simulink model "KD_cl_harness_cl_ouports_added"  (R2015b)
settings: Solver=ode45  StartTime=0  StopTime=inf  FixedStep=0.01  MaxStep=0.005  RelTol=1e-5  AbsTol=1e-5
undefined symbols (not defined in the file or in its folder): A2, bin_vec, c_0, c_1000, c_1000inv, c_100inv, c_1d2p4, c_1p7, c_4400inv, c_5500inv, c_80, c_compmap, c_ctok, c_fflow_max, c_fflow_min, c_filt, c_flowdiv, c_flowmin, c_flowmult, c_inf, c_km1d2k, c_n1, c_p00001, c_p01, c_p1e9, c_p4d1p4, c_pincomp, c_rair, c_roacorr, c_rpmtoradpers, c_svrthrottle1, c_svrthrottle2, c_svrthrottlearg, c_svrthrottlebeta, c_vnliftmax, c_vnliftmin, cl_offset, clff, Coefs, const, const_exhat, const_vec, Dual_array, dual_zero, egr_ecu_ff, expcon, f_mat, gs_jul, HQP_eps, HQP_INF, HQP_saturation, IV, L2, length_L, maxL, mHQP_saturation, minL, Newton, nRed, num_constraints ... (+22)
libraries: simulink x33
(part 3 of 6)

== system KD_cl_harness_cl_ouports_added/ctrl_rb_explicit_20140220_v6_simp/egr_est ==
  maf : Inport
  wcyl : Inport  Port=2
  ene : Inport  Port=3
  valve : Inport  Port=4
  Gain7 : Gain  Gain=100
      settings: AttributesFormatString=%<Gain>
  Product3 : Product  Inputs=**/  RndMeth=Zero
  Product4 : Product  Inputs=*/  RndMeth=Zero
  Saturation1 : Saturate  UpperLimit=c_inf  LowerLimit=c_0
      settings: AttributesFormatString=%<LowerLimit>\n%<UpperLimit>
  Saturation3 : Saturate  UpperLimit=c_inf  LowerLimit=c_p00001
      settings: AttributesFormatString=%<LowerLimit>\n%<UpperLimit>
  Sum11 : Sum  Inputs=+-|
  custom_filter : Subsystem  Tag=FilterWizardSubSystem
      settings: ErrorFcn=dspFilterRealizedInBasicElemsAlgLoopErrFcnCallback
  interp : Subsystem  Tag=FilterWizardSubSystem
      settings: ErrorFcn=dspFilterRealizedInBasicElemsAlgLoopErrFcnCallback
  mintos : Constant  Value=60  OutDataTypeStr=single
      settings: AttributesFormatString=%<Value>
  egrr : Outport
  wegr : Outport  Port=2
  wcylgps : Outport  Port=3
  sat_out-17 : Outport  Port=4
  sat_out-18 : Outport  Port=5
  sat_out-25 : Outport  Port=6
  sat_out-26 : Outport  Port=7
  wires:
  [MAF] -> Sum11/2
  Product3/1 -> interp/3(Wcyl)
  mintos/1 -> Product3/3
  Sum11/1 -> Saturation1/1, sat_out-17/1
  Product4/1 -> Gain7/1
  Gain7/1 -> egrr/1
  maf/1 -> [MAF]
  wcyl/1 -> Product3/1
  ene/1 -> Product3/2
  Saturation1/1 -> custom_filter/1(Input)
  Saturation3/1 -> Product4/2
  interp/1(Wcylhat) -> wcylgps/1, Sum11/1, [wcyl]
  [MAF] -> interp/2(MAF)
  valve/1 -> interp/1(valve)
  custom_filter/1(Output) -> Product4/1, wegr/1
  [wcyl] -> Saturation3/1, sat_out-18/1
  custom_filter/2(sat_out-25) -> sat_out-25/1
  custom_filter/3(sat_out-26) -> sat_out-26/1

== system KD_cl_harness_cl_ouports_added/ctrl_rb_explicit_20140220_v6_simp/gain_schechule ==
  ene : Inport
  qv : Inport  Port=2
  maprefadd1 : Lookup2D  RowIndex=gs_jul.rowsene  ColumnIndex=gs_jul.colsqv  Table=gs_jul.vegr  LookUpMeth=Interpolation-Use End Values
      settings: AttributesFormatString=%<LookUpMeth>\n%<RowIndex>\n%<ColumnIndex>\n%<Table>
  maprefadd2 : Lookup2D  RowIndex=gs_jul.rowsene  ColumnIndex=gs_jul.colsqv  Table=gs_jul.vgt  LookUpMeth=Interpolation-Use End Values
      settings: AttributesFormatString=%<LookUpMeth>\n%<RowIndex>\n%<ColumnIndex>\n%<Table>
  zero1 : Constant  Value=0  OutDataTypeStr=single  SampleTime=sample_time
      settings: AttributesFormatString=%<Value>\n%<SampleTime>
  zero15 : Constant  Value=0  OutDataTypeStr=single  SampleTime=sample_time
      settings: AttributesFormatString=%<Value>\n%<SampleTime>
  gs1 : Outport
  gs2 : Outport  Port=2
  gs3 : Outport  Port=3
  gs4 : Outport  Port=4
  wires:
  qv/1 -> [w_f]
  ene/1 -> [engine_speed_rpm]
  zero1/1 -> gs4/1
  zero15/1 -> gs3/1
  maprefadd1/1 -> gs2/1
  maprefadd2/1 -> gs1/1
  [engine_speed_rpm] -> maprefadd1/1
  [w_f] -> maprefadd1/2
  [engine_speed_rpm] -> maprefadd2/1
  [w_f] -> maprefadd2/2

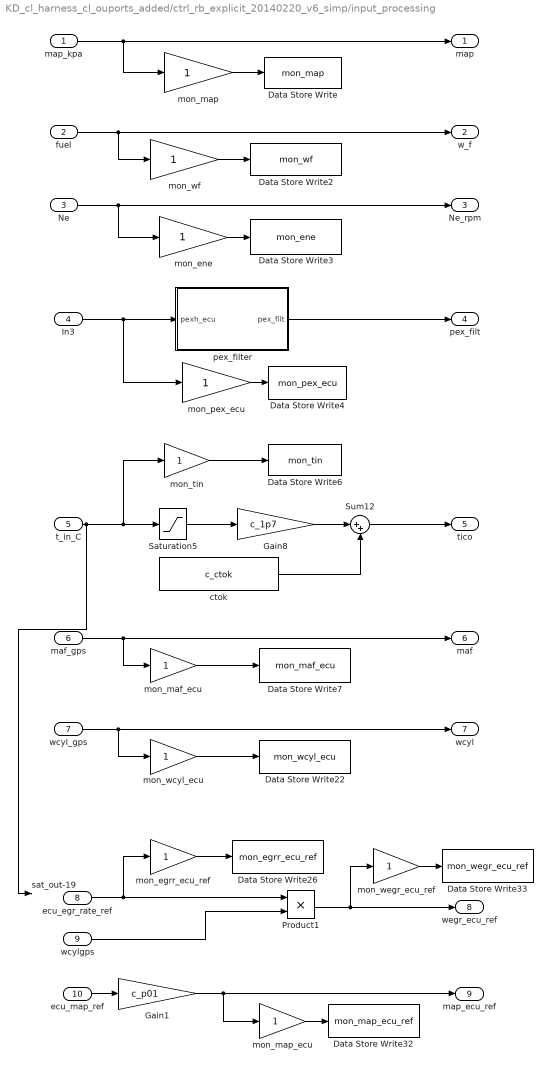
== system KD_cl_harness_cl_ouports_added/ctrl_rb_explicit_20140220_v6_simp/input_processing ==
  map_kpa : Inport
  fuel : Inport  Port=2
  Ne : Inport  Port=3
  In3 : Inport  Port=4
  t_in_C : Inport  Port=5
  maf_gps : Inport  Port=6
  wcyl_gps : Inport  Port=7
  ecu_egr_rate_ref : Inport  Port=8
  wcylgps : Inport  Port=9
  ecu_map_ref : Inport  Port=10
  Data Store Write : DataStoreWrite  DataStoreName=mon_map
  Data Store Write2 : DataStoreWrite  DataStoreName=mon_wf
  Data Store Write22 : DataStoreWrite  DataStoreName=mon_wcyl_ecu
  Data Store Write26 : DataStoreWrite  DataStoreName=mon_egrr_ecu_ref
  Data Store Write3 : DataStoreWrite  DataStoreName=mon_ene
  Data Store Write32 : DataStoreWrite  DataStoreName=mon_map_ecu_ref
  Data Store Write33 : DataStoreWrite  DataStoreName=mon_wegr_ecu_ref
  Data Store Write4 : DataStoreWrite  DataStoreName=mon_pex_ecu
  Data Store Write6 : DataStoreWrite  DataStoreName=mon_tin
  Data Store Write7 : DataStoreWrite  DataStoreName=mon_maf_ecu
  Gain1 : Gain  Gain=c_p01
      settings: AttributesFormatString=%<Gain>
  Gain8 : Gain  Gain=c_1p7
      settings: AttributesFormatString=%<Gain>
  Product1 : Product  RndMeth=Zero
  Saturation5 : Saturate  UpperLimit=c_inf  LowerLimit=c_0
      settings: AttributesFormatString=%<LowerLimit>\n%<UpperLimit>
  Sum12 : Sum  Inputs=|++
  ctok : Constant  Value=c_ctok  OutDataTypeStr=single  SampleTime=sample_time
      settings: AttributesFormatString=%<Value>\n%<SampleTime>
  mon_egrr_ecu_ref : Gain
  mon_ene : Gain
  mon_maf_ecu : Gain
  mon_map : Gain
  mon_map_ecu : Gain
  mon_pex_ecu : Gain
  mon_tin : Gain
  mon_wcyl_ecu : Gain
  mon_wegr_ecu_ref : Gain
  mon_wf : Gain
  pex_filter : Subsystem  SystemSampleTime=.016
  map : Outport
  w_f : Outport  Port=2
  Ne_rpm : Outport  Port=3
  pex_filt : Outport  Port=4
  tico : Outport  Port=5
  maf : Outport  Port=6
  wcyl : Outport  Port=7
  wegr_ecu_ref : Outport  Port=8
  map_ecu_ref : Outport  Port=9
  sat_out-19 : Outport  Port=10
  wires:
  Gain1/1 -> mon_map_ecu/1, map_ecu_ref/1
  Product1/1 -> mon_wegr_ecu_ref/1, wegr_ecu_ref/1
  mon_wegr_ecu_ref/1 -> Data Store Write33/1
  mon_map_ecu/1 -> Data Store Write32/1
  ecu_egr_rate_ref/1 -> Product1/1, mon_egrr_ecu_ref/1
  mon_egrr_ecu_ref/1 -> Data Store Write26/1
  In3/1 -> mon_pex_ecu/1, pex_filter/1(pexh_ecu)
  t_in_C/1 -> Saturation5/1, mon_tin/1, sat_out-19/1
  ctok/1 -> Sum12/2
  Gain8/1 -> Sum12/1
  Saturation5/1 -> Gain8/1
  mon_wf/1 -> Data Store Write2/1
  mon_ene/1 -> Data Store Write3/1
  mon_pex_ecu/1 -> Data Store Write4/1
  mon_tin/1 -> Data Store Write6/1
  mon_maf_ecu/1 -> Data Store Write7/1
  mon_wcyl_ecu/1 -> Data Store Write22/1
  fuel/1 -> w_f/1, mon_wf/1
  Ne/1 -> mon_ene/1, Ne_rpm/1
  maf_gps/1 -> mon_maf_ecu/1, maf/1
  wcyl_gps/1 -> wcyl/1, mon_wcyl_ecu/1
  pex_filter/1(pex_filt) -> pex_filt/1
  Sum12/1 -> tico/1
  wcylgps/1 -> Product1/2
  ecu_map_ref/1 -> Gain1/1
  map_kpa/1 -> mon_map/1, map/1
  mon_map/1 -> Data Store Write/1

== system KD_cl_harness_cl_ouports_added/ctrl_rb_explicit_20140220_v6_simp/invert_flow ==
  valve_flow_command : Inport
  ne_rpm : Inport  Port=2
  qv_mm3st : Inport  Port=3
  Saturation1 : Saturate  UpperLimit=150  LowerLimit=c_0
      settings: AttributesFormatString=%<LowerLimit>\n%<UpperLimit>
  d3inv : Lookup_n-D  NumberOfTableDimensions=3  BreakpointsForDimension1=valveinv.wegr_row  BreakpointsForDimension2=valveinv.ene_column  BreakpointsForDimension3=valveinv.fuel_z  Table=valveinv.valve  ExtrapMethod=Clip  UseLastTableValue=on  InputSameDT=on
      settings: AttributesFormatString=%<BreakpointsForDimension1>\n%<BreakpointsForDimension2>\n%<BreakpointsForDimension3>\n%<Table>\n%<UseLastTableValue>\n%<InterpMethod>
  togps : Gain  Gain=c_1000
      settings: AttributesFormatString=%<Gain>
  uvalve : Outport
  sat_out-20 : Outport  Port=2
  wires:
  Saturation1/1 -> uvalve/1
  d3inv/1 -> Saturation1/1, sat_out-20/1
  togps/1 -> d3inv/1
  qv_mm3st/1 -> d3inv/3
  ne_rpm/1 -> d3inv/2
  valve_flow_command/1 -> togps/1

== system KD_cl_harness_cl_ouports_added/ctrl_rb_explicit_20140220_v6_simp/ntremap ==
  u_EGR_throttle : Inport
  omega_engine_rpm : Inport  Port=2
  T_out_IC : Inport  Port=3
  maf : Inport  Port=4
  Data Store Read18 : DataStoreRead  DataStoreName=man_ntcons
  Divide6 : Product  Inputs=*/
  Saturation1 : Saturate  UpperLimit=50  LowerLimit=8
      settings: AttributesFormatString=%<LowerLimit>\n%<UpperLimit>
  Unit Delay3 : UnitDelay  SampleTime=-1
      settings: AttributesFormatString=%<X0>
  custom_filter : Subsystem  Tag=FilterWizardSubSystem
      settings: ErrorFcn=dspFilterRealizedInBasicElemsAlgLoopErrFcnCallback
  init : Constant  OutDataTypeStr=single  SampleTime=sample_time
      settings: AttributesFormatString=%<Value>\n%<SampleTime>
  man_ntcons : Gain
  remap_wt_to_map : Subsystem
  thousand : Constant  Value=1000  OutDataTypeStr=single  SampleTime=sample_time
      settings: AttributesFormatString=%<Value>\n%<SampleTime>
  mapconsremaped : Outport
  wtinv : Outport  Port=2
  sat_out-21 : Outport  Port=3
  sat_out-27 : Outport  Port=4
  sat_out-28 : Outport  Port=5
  sat_out-29 : Outport  Port=6
  sat_out-30 : Outport  Port=7
  sat_out-45 : Outport  Port=8
  sat_out-46 : Outport  Port=9
  sat_out-58 : Outport  Port=10
  sat_out-59 : Outport  Port=11
  sat_out-60 : Outport  Port=12
  sat_out-61 : Outport  Port=13
  sat_out-62 : Outport  Port=14
  sat_out-63 : Outport  Port=15
  sat_out-64 : Outport  Port=16
  sat_out-65 : Outport  Port=17
  out-17 : Outport  Port=18
  out-28 : Outport  Port=19
  wires:
  remap_wt_to_map/2(wtinv) -> wtinv/1
  Saturation1/1 -> remap_wt_to_map/4(In4)
  Data Store Read18/1 -> man_ntcons/1
  init/1 -> remap_wt_to_map/7(In7)
  remap_wt_to_map/1(pinv) -> mapconsremaped/1
  man_ntcons/1 -> Saturation1/1, sat_out-21/1
  u_EGR_throttle/1 -> Unit Delay3/1
  omega_engine_rpm/1 -> remap_wt_to_map/2(In2)
  T_out_IC/1 -> remap_wt_to_map/5(In5)
  custom_filter/1(Output) -> remap_wt_to_map/6(In6)
  Unit Delay3/1 -> remap_wt_to_map/1(In1)
  thousand/1 -> Divide6/2
  maf/1 -> Divide6/1
  Divide6/1 -> custom_filter/1(Input), remap_wt_to_map/3(In3)
  custom_filter/2(sat_out-27) -> sat_out-27/1
  custom_filter/3(sat_out-28) -> sat_out-28/1
  remap_wt_to_map/3(sat_out-29) -> sat_out-29/1
  remap_wt_to_map/4(sat_out-30) -> sat_out-30/1
  remap_wt_to_map/5(sat_out-45) -> sat_out-45/1
  remap_wt_to_map/6(sat_out-46) -> sat_out-46/1
  remap_wt_to_map/7(sat_out-58) -> sat_out-58/1
  remap_wt_to_map/8(sat_out-59) -> sat_out-59/1
  remap_wt_to_map/9(sat_out-60) -> sat_out-60/1
  remap_wt_to_map/10(sat_out-61) -> sat_out-61/1
  remap_wt_to_map/11(sat_out-62) -> sat_out-62/1
  remap_wt_to_map/12(sat_out-63) -> sat_out-63/1
  remap_wt_to_map/13(sat_out-64) -> sat_out-64/1
  remap_wt_to_map/14(sat_out-65) -> sat_out-65/1
  remap_wt_to_map/15(out-17) -> out-17/1
  remap_wt_to_map/16(out-28) -> out-28/1

== system KD_cl_harness_cl_ouports_added/ctrl_rb_explicit_20140220_v6_simp/pex_estimator ==
  valvez : Inport
  Ne_rpm : Inport  Port=2
  map : Inport  Port=3
  wegr : Inport  Port=4
  tico : Inport  Port=5
  pex_filt : Inport  Port=6
  while : Inport  Port=7
  Data Store Write21 : DataStoreWrite  DataStoreName=mon_pex_hat
  Unit Delay2 : UnitDelay  InitialCondition=200  SampleTime=-1
      settings: AttributesFormatString=%<X0>
  WhileIteratorSubsystem : Subsystem  TreatAsAtomicUnit=on
  mon_pex_hat : Gain
  pex_hat : Outport
  dwdp : Outport  Port=2
  pex_hat_limited : Outport  Port=3
  sat_out-31 : Outport  Port=4
  sat_out-32 : Outport  Port=5
  sat_out-33 : Outport  Port=6
  sat_out-34 : Outport  Port=7
  sat_out-35 : Outport  Port=8
  sat_out-36 : Outport  Port=9
  sat_out-47 : Outport  Port=10
  sat_out-48 : Outport  Port=11
  sat_out-49 : Outport  Port=12
  sat_out-50 : Outport  Port=13
  sat_out-51 : Outport  Port=14
  sat_out-52 : Outport  Port=15
  sat_out-53 : Outport  Port=16
  sat_out-54 : Outport  Port=17
  sat_out-55 : Outport  Port=18
  sat_out-56 : Outport  Port=19
  sat_out-57 : Outport  Port=20
  wires:
  WhileIteratorSubsystem/3(pex_limited) -> mon_pex_hat/1, Unit Delay2/1, pex_hat_limited/1
  mon_pex_hat/1 -> Data Store Write21/1
  Unit Delay2/1 -> WhileIteratorSubsystem/8(pexz)
  valvez/1 -> WhileIteratorSubsystem/1(valvez)
  Ne_rpm/1 -> WhileIteratorSubsystem/2(Ne_rpm)
  WhileIteratorSubsystem/1(pex) -> pex_hat/1
  map/1 -> WhileIteratorSubsystem/3(map)
  wegr/1 -> WhileIteratorSubsystem/4(wger)
  tico/1 -> WhileIteratorSubsystem/5(tico)
  WhileIteratorSubsystem/2(dwdp) -> dwdp/1
  pex_filt/1 -> WhileIteratorSubsystem/6(pex_filt)
  while/1 -> WhileIteratorSubsystem/7(While)
  WhileIteratorSubsystem/4(sat_out-31) -> sat_out-31/1
  WhileIteratorSubsystem/5(sat_out-32) -> sat_out-32/1
  WhileIteratorSubsystem/6(sat_out-33) -> sat_out-33/1
  WhileIteratorSubsystem/7(sat_out-34) -> sat_out-34/1
  WhileIteratorSubsystem/8(sat_out-35) -> sat_out-35/1
  WhileIteratorSubsystem/9(sat_out-36) -> sat_out-36/1
  WhileIteratorSubsystem/10(sat_out-47) -> sat_out-47/1
  WhileIteratorSubsystem/11(sat_out-48) -> sat_out-48/1
  WhileIteratorSubsystem/12(sat_out-49) -> sat_out-49/1
  WhileIteratorSubsystem/13(sat_out-50) -> sat_out-50/1
  WhileIteratorSubsystem/14(sat_out-51) -> sat_out-51/1
  WhileIteratorSubsystem/15(sat_out-52) -> sat_out-52/1
  WhileIteratorSubsystem/16(sat_out-53) -> sat_out-53/1
  WhileIteratorSubsystem/17(sat_out-54) -> sat_out-54/1
  WhileIteratorSubsystem/18(sat_out-55) -> sat_out-55/1
  WhileIteratorSubsystem/19(sat_out-56) -> sat_out-56/1
  WhileIteratorSubsystem/20(sat_out-57) -> sat_out-57/1

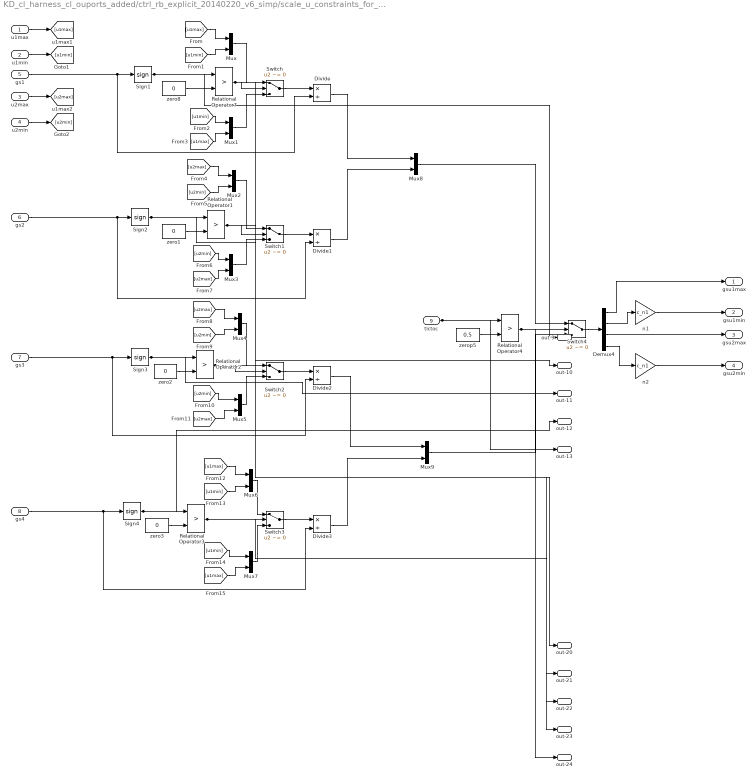
== system KD_cl_harness_cl_ouports_added/ctrl_rb_explicit_20140220_v6_simp/scale_u_constraints_for_gs ==
  u1max : Inport
  u1min : Inport  Port=2
  u2max : Inport  Port=3
  u2min : Inport  Port=4
  gs1 : Inport  Port=5
  gs2 : Inport  Port=6
  gs3 : Inport  Port=7
  gs4 : Inport  Port=8
  tictoc : Inport  Port=9
  Demux4 : Demux
  Divide{,1..3} (4 alike) : Product  Inputs=*/
  Mux{,1..9} (10 alike) : Mux  Inputs=2
  Relational Operator{1..4,7} (5 alike) : RelationalOperator  Operator=>  OutDataTypeStr=boolean
      settings: AttributesFormatString=%<Operator>
  Sign{1..4} (4 alike) : Signum
  Switch{,1..4} (5 alike) : Switch  Criteria=u2 ~= 0
      settings: AttributesFormatString=%<Criteria>
  n1 : Gain  Gain=c_n1
      settings: AttributesFormatString=%<Gain>
  n2 : Gain  Gain=c_n1
      settings: AttributesFormatString=%<Gain>
  zero{1..3,8} (4 alike) : Constant  Value=0  OutDataTypeStr=single  SampleTime=sample_time
      settings: AttributesFormatString=%<Value>\n%<SampleTime>
  zerop5 : Constant  Value=0.5  OutDataTypeStr=single  SampleTime=sample_time
      settings: AttributesFormatString=%<Value>\n%<SampleTime>
  gsu1max : Outport
  gsu1min : Outport  Port=2
  gsu2max : Outport  Port=3
  gsu2min : Outport  Port=4
  out-9 : Outport  Port=5
  out-10 : Outport  Port=6
  out-11 : Outport  Port=7
  out-12 : Outport  Port=8
  out-13 : Outport  Port=9
  out-20 : Outport  Port=10
  out-21 : Outport  Port=11
  out-22 : Outport  Port=12
  out-23 : Outport  Port=13
  out-24 : Outport  Port=14
  wires:
  n2/1 -> gsu2min/1
  n1/1 -> gsu1min/1
  Demux4/4 -> n2/1
  Demux4/3 -> gsu2max/1
  Demux4/2 -> n1/1
  Demux4/1 -> gsu1max/1
  Switch4/1 -> Demux4/1
  Mux9/1 -> Switch4/3
  Mux8/1 -> Switch4/1
  Divide3/1 -> Mux9/2
  Divide2/1 -> Mux9/1
  Divide1/1 -> Mux8/2
  Divide/1 -> Mux8/1
  gs4/1 -> Sign4/1, Divide3/2
  Switch3/1 -> Divide3/1
  Mux6/1 -> Switch3/1
  Mux7/1 -> Switch3/3
  [u1max] -> Mux7/2
  [u1min] -> Mux7/1
  [u1min] -> Mux6/2
  [u1max] -> Mux6/1
  gs3/1 -> Divide2/2, Sign3/1
  Switch2/1 -> Divide2/1
  Mux4/1 -> Switch2/1
  Mux5/1 -> Switch2/3
  [u2max] -> Mux5/2
  [u2min] -> Mux5/1
  [u2min] -> Mux4/2
  [u2max] -> Mux4/1
  gs2/1 -> Sign2/1, Divide1/2
  Switch1/1 -> Divide1/1
  Mux2/1 -> Switch1/1
  Mux3/1 -> Switch1/3
  [u2max] -> Mux3/2
  [u2min] -> Mux3/1
  [u2min] -> Mux2/2
  [u2max] -> Mux2/1
  u2min/1 -> [u2min]
  u2max/1 -> [u2max]
  gs1/1 -> Sign1/1, Divide/2
  Switch/1 -> Divide/1
  Mux/1 -> Switch/1
  Mux1/1 -> Switch/3
  [u1max] -> Mux1/2
  [u1min] -> Mux1/1
  [u1min] -> Mux/2
  [u1max] -> Mux/1
  u1min/1 -> [u1min]
  u1max/1 -> [u1max]
  zero8/1 -> Relational Operator7/2
  Sign1/1 -> Relational Operator7/1, out-9/1
  Relational Operator7/1 -> Switch/2, out-20/1
  zero1/1 -> Relational Operator1/2
  Sign2/1 -> Relational Operator1/1, out-10/1
  Relational Operator1/1 -> Switch1/2, out-21/1
  zero2/1 -> Relational Operator2/2
  Sign3/1 -> Relational Operator2/1, out-11/1
  Relational Operator2/1 -> Switch2/2, out-22/1
  zero3/1 -> Relational Operator3/2
  Sign4/1 -> Relational Operator3/1, out-12/1
  Relational Operator3/1 -> Switch3/2, out-23/1
  zerop5/1 -> Relational Operator4/2
  tictoc/1 -> Relational Operator4/1, out-13/1
  Relational Operator4/1 -> Switch4/2, out-24/1

== system KD_cl_harness_cl_ouports_added/ctrl_rb_explicit_20140220_v6_simp/scheduled_observer ==
  tictoc : Inport
  map : Inport  Port=2
  egrr : Inport  Port=3
  xhatROpm1 : Inport  Port=4
  u : Inport  Port=5
  If : If  IfExpression=u1 > 0.5  ShowElse=off
  observer : Subsystem
  xhatRO : Outport
  xhat : Outport  Port=2
  wires:
  If/1 -> observer/Action
  tictoc/1 -> If/1
  observer/1(xhatRO) -> xhatRO/1
  observer/2(xhat) -> xhat/1
  map/1 -> observer/1(map)
  egrr/1 -> observer/2(egrr)
  xhatROpm1/1 -> observer/3(xhatROpm)
  u/1 -> observer/4(u)

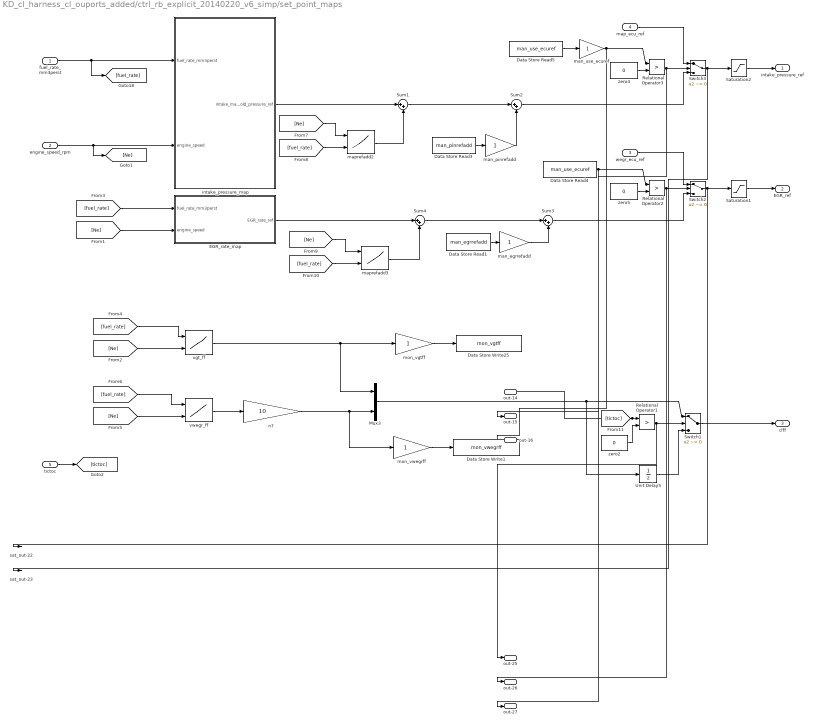
== system KD_cl_harness_cl_ouports_added/ctrl_rb_explicit_20140220_v6_simp/set_point_maps ==
  fuel_rate_mm3perst : Inport
  engine_speed_rpm : Inport  Port=2
  wegr_ecu_ref : Inport  Port=3
  map_ecu_ref : Inport  Port=4
  tictoc : Inport  Port=5
  Data Store Read1 : DataStoreRead  DataStoreName=man_egrrefadd
  Data Store Read3 : DataStoreRead  DataStoreName=man_pinrefadd
  Data Store Read4 : DataStoreRead  DataStoreName=man_use_ecuref
  Data Store Read5 : DataStoreRead  DataStoreName=man_use_ecuref
  Data Store Write1 : DataStoreWrite  DataStoreName=mon_vwegrff
  Data Store Write25 : DataStoreWrite  DataStoreName=mon_vgtff
  EGR_rate_map : Subsystem
  Mux3 : Mux  Inputs=2
  Relational Operator1 : RelationalOperator  Operator=>  OutDataTypeStr=boolean
      settings: AttributesFormatString=%<Operator>
  Relational Operator2 : RelationalOperator  Operator=>  OutDataTypeStr=boolean
      settings: AttributesFormatString=%<Operator>
  Relational Operator3 : RelationalOperator  Operator=>  OutDataTypeStr=boolean
      settings: AttributesFormatString=%<Operator>
  Saturation1 : Saturate  UpperLimit=c_inf  LowerLimit=c_0
      settings: AttributesFormatString=%<LowerLimit>\n%<UpperLimit>
  Saturation2 : Saturate  UpperLimit=c_inf  LowerLimit=90
      settings: AttributesFormatString=%<LowerLimit>\n%<UpperLimit>
  Sum{1..4} (4 alike) : Sum  Inputs=|++
  Switch1 : Switch  Criteria=u2 ~= 0
      settings: AttributesFormatString=%<Criteria>
  Switch2 : Switch  Criteria=u2 ~= 0
      settings: AttributesFormatString=%<Criteria>
  Switch3 : Switch  Criteria=u2 ~= 0
      settings: AttributesFormatString=%<Criteria>
  Unit Delay5 : UnitDelay  InitialCondition=[40;0]  SampleTime=-1
      settings: AttributesFormatString=%<X0>
  intake_pressure_map : Subsystem
  man_egrrefadd : Gain
  man_pinrefadd : Gain
  man_use_ecuref : Gain
  maprefadd2 : Lookup2D  RowIndex=cl_offset.rowsene  ColumnIndex=cl_offset.colsqv  Table=cl_offset.map  LookUpMeth=Interpolation-Use End Values
      settings: AttributesFormatString=%<LookUpMeth>\n%<RowIndex>\n%<ColumnIndex>\n%<Table>
  maprefadd3 : Lookup2D  RowIndex=cl_offset.rowsene  ColumnIndex=cl_offset.colsqv  Table=cl_offset.wegr  LookUpMeth=Interpolation-Use End Values
      settings: AttributesFormatString=%<LookUpMeth>\n%<RowIndex>\n%<ColumnIndex>\n%<Table>
  mon_vgtff : Gain
  mon_vwegrff : Gain
  n7 : Gain  Gain=10
      settings: AttributesFormatString=%<Gain>
  vgt_ff : Lookup2D  RowIndex=clff.rowsqv  ColumnIndex=clff.colsene  Table=clff.vgt  LookUpMeth=Interpolation-Use End Values
      settings: AttributesFormatString=%<LookUpMeth>\n%<RowIndex>\n%<ColumnIndex>\n%<Table>
  vwegr_ff : Lookup2D  RowIndex=clff.rowsqv  ColumnIndex=clff.colsene  Table=clff.vwegr  LookUpMeth=Interpolation-Use End Values
      settings: AttributesFormatString=%<LookUpMeth>\n%<RowIndex>\n%<ColumnIndex>\n%<Table>
  zero2 : Constant  Value=0  OutDataTypeStr=single  SampleTime=sample_time
      settings: AttributesFormatString=%<Value>\n%<SampleTime>
  zero4 : Constant  Value=0  OutDataTypeStr=single  SampleTime=sample_time
      settings: AttributesFormatString=%<Value>\n%<SampleTime>
  zero5 : Constant  Value=0  OutDataTypeStr=single  SampleTime=sample_time
      settings: AttributesFormatString=%<Value>\n%<SampleTime>
  intake_pressure_ref : Outport
  EGR_ref : Outport  Port=2
  clff : Outport  Port=3
  sat_out-22 : Outport  Port=4
  sat_out-23 : Outport  Port=5
  out-14 : Outport  Port=6
  out-15 : Outport  Port=7
  out-16 : Outport  Port=8
  out-25 : Outport  Port=9
  out-26 : Outport  Port=10
  out-27 : Outport  Port=11
  wires:
  mon_vwegrff/1 -> Data Store Write1/1
  mon_vgtff/1 -> Data Store Write25/1
  Switch3/1 -> Saturation2/1, sat_out-23/1
  map_ecu_ref/1 -> Switch3/1
  Sum2/1 -> Switch3/3
  Relational Operator3/1 -> Switch3/2, out-27/1
  Data Store Read5/1 -> man_use_ecuref/1
  zero4/1 -> Relational Operator3/2
  man_use_ecuref/1 -> Relational Operator3/1, out-16/1
  wegr_ecu_ref/1 -> Switch2/1
  Switch2/1 -> Saturation1/1, sat_out-22/1
  Sum3/1 -> Switch2/3
  Relational Operator2/1 -> Switch2/2, out-26/1
  Data Store Read4/1 -> Relational Operator2/1, out-15/1
  zero5/1 -> Relational Operator2/2
  Saturation2/1 -> intake_pressure_ref/1
  [fuel_rate] -> maprefadd3/2
  Sum4/1 -> Sum3/1
  EGR_rate_map/1(EGR_rate_ref) -> Sum4/1
  maprefadd3/1 -> Sum4/2
  [Ne] -> maprefadd3/1
  [Ne] -> maprefadd2/1
  [fuel_rate] -> maprefadd2/2
  maprefadd2/1 -> Sum1/2
  Sum1/1 -> Sum2/1
  intake_pressure_map/1(intake_manifold_pressure_ref) -> Sum1/1
  [Ne] -> EGR_rate_map/2(engine_speed)
  [fuel_rate] -> EGR_rate_map/1(fuel_rate_mm3perst)
  fuel_rate_mm3perst/1 -> intake_pressure_map/1(fuel_rate_mm3perst), [fuel_rate]
  engine_speed_rpm/1 -> [Ne], intake_pressure_map/2(engine_speed)
  Saturation1/1 -> EGR_ref/1
  Data Store Read3/1 -> man_pinrefadd/1
  Data Store Read1/1 -> man_egrrefadd/1
  man_pinrefadd/1 -> Sum2/2
  man_egrrefadd/1 -> Sum3/2
  [fuel_rate] -> vgt_ff/1
  [Ne] -> vgt_ff/2
  [fuel_rate] -> vwegr_ff/1
  [Ne] -> vwegr_ff/2
  vgt_ff/1 -> mon_vgtff/1, Mux3/1
  vwegr_ff/1 -> n7/1
  n7/1 -> Mux3/2, mon_vwegrff/1
  tictoc/1 -> [tictoc]
  Mux3/1 -> Switch1/1, Unit Delay5/1
  Relational Operator1/1 -> Switch1/2, out-25/1
  Unit Delay5/1 -> Switch1/3
  zero2/1 -> Relational Operator1/2
  [tictoc] -> Relational Operator1/1, out-14/1
  Switch1/1 -> clff/1

== system KD_cl_harness_cl_ouports_added/ctrl_rb_explicit_20140220_v6_simp/shift_x_hat ==
  map_ref : Inport
  x_hat : Inport  Port=2
  egr_ref : Inport  Port=3
  pex_hat : Inport  Port=4
  Data Store Write10 : DataStoreWrite  DataStoreName=mon_map_hat
  Data Store Write11 : DataStoreWrite  DataStoreName=mon_egrr_hat
  Data Store Write12 : DataStoreWrite  DataStoreName=mon_x1_hat
  Demux3 : Demux  Outputs=[size(expcon.RobsA,1) 1 1]
  Mux2 : Mux  Inputs=5
  Sum8 : Sum  Inputs=-+|
  Sum9 : Sum  Inputs=-+|
  dummy : Constant  OutDataTypeStr=single  SampleTime=sample_time
      settings: AttributesFormatString=%<Value>\n%<SampleTime>
  mon_egrr_hat : Gain
  mon_map_hat : Gain
  mon_x1_hat : Gain
  x_hat_shift : Outport
  wires:
  Sum9/1 -> Mux2/3
  Sum8/1 -> Mux2/2
  Demux3/3 -> Sum9/2, mon_egrr_hat/1
  Demux3/2 -> Sum8/2, mon_map_hat/1
  Demux3/1 -> Mux2/1, mon_x1_hat/1
  mon_x1_hat/1 -> Data Store Write12/1
  mon_map_hat/1 -> Data Store Write10/1
  mon_egrr_hat/1 -> Data Store Write11/1
  dummy/1 -> Mux2/5
  map_ref/1 -> Sum8/1
  x_hat/1 -> Demux3/1
  egr_ref/1 -> Sum9/1
  Mux2/1 -> x_hat_shift/1
  pex_hat/1 -> Mux2/4

== system KD_cl_harness_cl_ouports_added/ctrl_rb_explicit_20140220_v6_simp/tictoc ==
  Lookup Table : Lookup  InputValues=[0 .25 .5 1]  Table=[1 1 0 0]  LookUpMeth=Interpolation-Use End Values  OutDataTypeStr=single
      settings: AttributesFormatString=%<LookUpMeth>
  Unit Delay16 : UnitDelay  InitialCondition=1  SampleTime=-1
      settings: AttributesFormatString=%<X0>
  tictoc : Outport
  wires:
  Unit Delay16/1 -> Lookup Table/1
  Lookup Table/1 -> Unit Delay16/1, tictoc/1

== system KD_cl_harness_cl_ouports_added/ctrl_rb_explicit_20140220_v6_simp/u_limits ==
  clff : Inport
  uz : Inport  Port=2
  flow_max : Inport  Port=3
  flow_min : Inport  Port=4
  Data Store Read26 : DataStoreRead  DataStoreName=man_vgt_max
  Demux4 : Demux  Outputs=2
  Saturation1 : Saturate  UpperLimit=95  LowerLimit=c_vnliftmin
      settings: AttributesFormatString=%<LowerLimit>\n%<UpperLimit>
  Sum13 : Sum  Inputs=++|
  Sum2 : Sum  Inputs=-+|  OutDataTypeStr=single
  Sum3 : Sum  Inputs=-+|
  Sum4 : Sum  Inputs=-+|  OutDataTypeStr=single
  Sum5 : Sum  Inputs=-+|  OutDataTypeStr=single
  man_vgt_max : Gain
  n3 : Gain  Gain=c_flowmult
      settings: AttributesFormatString=%<Gain>
  vnliftmin : Constant  Value=c_vnliftmin  OutDataTypeStr=single  SampleTime=sample_time
      settings: AttributesFormatString=%<Value>\n%<SampleTime>
  u1max : Outport
  u1min : Outport  Port=2
  u2max : Outport  Port=3
  u2min : Outport  Port=4
  sat_out-24 : Outport  Port=5
  wires:
  man_vgt_max/1 -> Saturation1/1, sat_out-24/1
  Data Store Read26/1 -> man_vgt_max/1
  Saturation1/1 -> Sum2/2
  Demux4/1 -> Sum3/1, Sum2/1
  vnliftmin/1 -> Sum3/2
  n3/1 -> Sum4/2
  Demux4/2 -> Sum5/1, Sum4/1
  Sum13/1 -> Demux4/1
  flow_min/1 -> Sum5/2
  Sum2/1 -> u1max/1
  clff/1 -> Sum13/1
  Sum3/1 -> u1min/1
  uz/1 -> Sum13/2
  Sum4/1 -> u2max/1
  flow_max/1 -> n3/1
  Sum5/1 -> u2min/1

== system KD_cl_harness_cl_ouports_added/pre-throttle manifold/p_preThrottle ==
  W_compressor : Inport
  W_throttle : Inport  Port=2
  T_out_compressor : Inport  Port=3
  T_out_IC_data : Inport  Port=4
  Cus_integrator : Subsystem
  Fcn1 : Fcn  Expr=u(4)*(u(1) - u(2))
  Mux : Mux
  gamma*R/V_preThrottle : Gain  Gain=const.gamma_air*const.R_specific_air_KJ_per_kg_kelvin/Coefs.V_prethrottle_m3
  "p_pre_throttle " : Outport
  wires:
  Cus_integrator/1(p_preThrottle) -> "p_pre_throttle "/1
  gamma*R/V_preThrottle/1 -> Cus_integrator/1(in)
  Fcn1/1 -> gamma*R/V_preThrottle/1
  Mux/1 -> Fcn1/1
  W_compressor/1 -> Mux/1
  W_throttle/1 -> Mux/2
  T_out_compressor/1 -> Mux/3
  T_out_IC_data/1 -> Mux/4

== system KD_cl_harness_cl_ouports_added/steps/Subsystem ==
  In1 : Inport
  Rate Limiter : RateLimiter  RisingSlewLimit=22  FallingSlewLimit=-22  SampleTimeMode=inherited  InitialCondition=30
  Unit Delay : UnitDelay  InitialCondition=30  SampleTime=-1
  Out1 : Outport
  wires:
  In1/1 -> Unit Delay/1
  Unit Delay/1 -> Rate Limiter/1
  Rate Limiter/1 -> Out1/1

== system KD_cl_harness_cl_ouports_added/steps/Subsystem1 ==
  In1 : Inport
  Rate Limiter : RateLimiter  RisingSlewLimit=1000  FallingSlewLimit=-1000  SampleTimeMode=inherited  InitialCondition=2500
  Unit Delay : UnitDelay  InitialCondition=2500  SampleTime=-1
  Out1 : Outport
  wires:
  Rate Limiter/1 -> Out1/1
  Unit Delay/1 -> Rate Limiter/1
  In1/1 -> Unit Delay/1

== system KD_cl_harness_cl_ouports_added/steps/Subsystem2 ==
  In1 : Inport
  Rate Limiter : RateLimiter  RisingSlewLimit=22  FallingSlewLimit=-22  SampleTimeMode=inherited  InitialCondition=5
  Unit Delay : UnitDelay  InitialCondition=5  SampleTime=-1
  Out1 : Outport
  wires:
  Rate Limiter/1 -> Out1/1
  Unit Delay/1 -> Rate Limiter/1
  In1/1 -> Unit Delay/1

== system KD_cl_harness_cl_ouports_added/EGR Throttle/EGR Throttle/Throttle Model2 ==
  TA[deg] : Inport
  Ne[rpm] : Inport  Port=2
  Pim[Pa] : Inport  Port=3
  Tim[K] : Inport  Port=4
  Pamb[Pa] : Inport  Port=5
  Tamb[K] : Inport  Port=6
  Air Model_map_use : Subsystem
  Ra : Constant  Value=const.Rair
  mt[kg/sec] : Outport
  forwardmt[kg/sec] : Outport  Port=2
  backwardmt[kg/sec] : Outport  Port=3
  sat_out-37 : Outport  Port=4
  sat_out-38 : Outport  Port=5
  sat_out-39 : Outport  Port=6
  sat_out-40 : Outport  Port=7
  out-1 : Outport  Port=8
  out-3 : Outport  Port=9
  out-4 : Outport  Port=10
  wires:
  TA[deg]/1 -> Air Model_map_use/1(TA[deg])
  Pamb[Pa]/1 -> Air Model_map_use/5(Pa[Pa])
  Tamb[K]/1 -> Air Model_map_use/6(Ta[K])
  Pim[Pa]/1 -> Air Model_map_use/3(Pim[Pa])
  Tim[K]/1 -> Air Model_map_use/4(Tim[K])
  Air Model_map_use/1(mt[kg/sec]) -> mt[kg/sec]/1
  Ra/1 -> Air Model_map_use/7(R_im), Air Model_map_use/8(R_a)
  Air Model_map_use/2(forwardmt) -> forwardmt[kg/sec]/1
  Ne[rpm]/1 -> Air Model_map_use/2(Ne[rpm])
  Air Model_map_use/3(backwardmt) -> backwardmt[kg/sec]/1
  Air Model_map_use/4(sat_out-37) -> sat_out-37/1
  Air Model_map_use/5(sat_out-38) -> sat_out-38/1
  Air Model_map_use/6(sat_out-39) -> sat_out-39/1
  Air Model_map_use/7(sat_out-40) -> sat_out-40/1
  Air Model_map_use/8(out-1) -> out-1/1
  Air Model_map_use/9(out-3) -> out-3/1
  Air Model_map_use/10(out-4) -> out-4/1

== system KD_cl_harness_cl_ouports_added/EGR Valve/SVR EGR/EGR_model ==
  TA[deg] : Inport
  Ne[rpm] : Inport  Port=2
  Pim[Pa] : Inport  Port=3
  Tim[K] : Inport  Port=4
  Pamb[Pa] : Inport  Port=5
  Tamb[K] : Inport  Port=6
  Air Model_map_use : Subsystem
  Ra : Constant  Value=const.Rair
  mt[kg/sec] : Outport
  forwardmt[kg/sec] : Outport  Port=2
  sat_out-41 : Outport  Port=3
  sat_out-42 : Outport  Port=4
  sat_out-43 : Outport  Port=5
  sat_out-44 : Outport  Port=6
  out-2 : Outport  Port=7
  out-5 : Outport  Port=8
  out-6 : Outport  Port=9
  wires:
  Ne[rpm]/1 -> Air Model_map_use/2(Ne[rpm])
  Air Model_map_use/2(forwardmt) -> forwardmt[kg/sec]/1
  Ra/1 -> Air Model_map_use/8(R_a), Air Model_map_use/7(R_im)
  Air Model_map_use/1(mt[kg/sec]) -> mt[kg/sec]/1
  Tim[K]/1 -> Air Model_map_use/4(Tim[K])
  Pim[Pa]/1 -> Air Model_map_use/3(Pim[Pa])
  Tamb[K]/1 -> Air Model_map_use/6(Ta[K])
  Pamb[Pa]/1 -> Air Model_map_use/5(Pa[Pa])
  TA[deg]/1 -> Air Model_map_use/1(TA[deg])
  Air Model_map_use/3(sat_out-41) -> sat_out-41/1
  Air Model_map_use/4(sat_out-42) -> sat_out-42/1
  Air Model_map_use/5(sat_out-43) -> sat_out-43/1
  Air Model_map_use/6(sat_out-44) -> sat_out-44/1
  Air Model_map_use/7(out-2) -> out-2/1
  Air Model_map_use/8(out-5) -> out-5/1
  Air Model_map_use/9(out-6) -> out-6/1

== system KD_cl_harness_cl_ouports_added/Exhaust Manifold/Exhaust Manifold/Cus_integrator ==
  in : Inport
  Integrator : Integrator  InitialCondition=IV.rho_exhaust_man  UpperSaturationLimit=maxL.rho_exhaust_man  LowerSaturationLimit=minL.rho_exhaust_man
  rho_exhaust : Outport
  wires:
  in/1 -> Integrator/1
  Integrator/1 -> rho_exhaust/1

== system KD_cl_harness_cl_ouports_added/Exhaust Manifold/Exhaust Manifold/Cus_integrator1 ==
  in : Inport
  Integrator1 : Integrator  InitialCondition=IV.F_exhaust  UpperSaturationLimit=maxL.F_exhuast_man  LowerSaturationLimit=minL.F_exhuast_man
  F2_exhaust : Outport
  wires:
  in/1 -> Integrator1/1
  Integrator1/1 -> F2_exhaust/1

== system KD_cl_harness_cl_ouports_added/Exhaust Manifold/Exhaust Manifold/Cus_integrator2 ==
  in : Inport
  Integrator2 : Integrator  InitialCondition=IV.p_exhaust_man  UpperSaturationLimit=maxL.p_exhaust_man  LowerSaturationLimit=minL.p_exhaust_man
  p_exhaust : Outport
  wires:
  Integrator2/1 -> p_exhaust/1
  in/1 -> Integrator2/1

== system KD_cl_harness_cl_ouports_added/Intake Manifold/Intake_manifold/Cus_integrator ==
  in : Inport
  Integrator : Integrator  InitialCondition=IV.rho_intake_man  UpperSaturationLimit=maxL.rho_intake_man  LowerSaturationLimit=minL.rho_intake_man
  rho_intake : Outport
  wires:
  in/1 -> Integrator/1
  Integrator/1 -> rho_intake/1

== system KD_cl_harness_cl_ouports_added/Intake Manifold/Intake_manifold/Cus_integrator1 ==
  in : Inport
  Integrator : Integrator  InitialCondition=IV.F_intake  UpperSaturationLimit="maxL.F1_intake_man   + 0.00001"  LowerSaturationLimit=minL.F1_intake_man
  F1_intake : Outport
  wires:
  in/1 -> Integrator/1
  Integrator/1 -> F1_intake/1

== system KD_cl_harness_cl_ouports_added/Intake Manifold/Intake_manifold/Cus_integrator2 ==
  in : Inport
  Integrator1 : Integrator  InitialCondition=IV.p_intake_man  UpperSaturationLimit=maxL.p_intake_man  LowerSaturationLimit=minL.p_intake_man
  p_intake : Outport
  wires:
  in/1 -> Integrator1/1
  Integrator1/1 -> p_intake/1

== system KD_cl_harness_cl_ouports_added/Turbo Rotational Dynamics/Turbo rot/Cus_integrator ==
  delta_torque : Inport
  Integrator1 : Integrator  InitialCondition=IV.omega_turbo_rads  UpperSaturationLimit=maxL.omega_turbo_rs  LowerSaturationLimit=minL.omega_turbo_rs
  NT_radS : Outport
  wires:
  delta_torque/1 -> Integrator1/1
  Integrator1/1 -> NT_radS/1

== system KD_cl_harness_cl_ouports_added/ctrl_rb_explicit_20140220_v6_simp/HQPKWIK_V6/QPKWIK_Main ==
  b : Inport
  x0 : Inport  Port=2
  c : Inport  Port=3
  Consraint matrix : Constant  Value=A2  VectorParams1D=off  OutDataTypeStr=single
      settings: AttributesFormatString=%<Value>\n%<VectorParams1D>
  IC_while_loop : Constant  OutDataTypeStr=boolean
      settings: AttributesFormatString=%<Value>
  QPKWIK_While_Loop : Subsystem
  const_vec : Constant  Value=const_vec  VectorParams1D=off  OutDataTypeStr=single
      settings: AttributesFormatString=%<Value>\n%<VectorParams1D>
  epsilon : Constant  Value=HQP_eps  VectorParams1D=off  OutDataTypeStr=single
      settings: AttributesFormatString=%<Value>\n%<VectorParams1D>
  controlinput : Outport
  SL_sum : Outport  Port=2  InitialOutput=0
  wires:
  QPKWIK_While_Loop/2(active_SL) -> SL_sum/1
  c/1 -> QPKWIK_While_Loop/7(c)
  epsilon/1 -> QPKWIK_While_Loop/3(In3)
  x0/1 -> QPKWIK_While_Loop/6(x0)
  IC_while_loop/1 -> QPKWIK_While_Loop/5(In5)
  b/1 -> QPKWIK_While_Loop/2(In2)
  const_vec/1 -> QPKWIK_While_Loop/4(In4)
  Consraint matrix/1 -> QPKWIK_While_Loop/1(In1)
  QPKWIK_While_Loop/1(x) -> controlinput/1

== system KD_cl_harness_cl_ouports_added/ctrl_rb_explicit_20140220_v6_simp/HQPKWIK_V6/b_extraction ==
  uinput : Inport
  Add : Sum  Inputs=+-
  Add1 : Sum  Inputs=+-
  Gain7 : Gain  Gain=-1
  MathFunction : Math  Operator=transpose  SaturateOnIntegerOverflow=on
  MathFunction1 : Math  Operator=transpose  SaturateOnIntegerOverflow=on
  MathFunction2 : Math  Operator=transpose  SaturateOnIntegerOverflow=on
  Product3 : Product  Multiplication=Matrix(*)  RndMeth=Zero
  Product4 : Product  Multiplication=Matrix(*)  RndMeth=Zero
  Reshape_input : Reshape  OutputDimensionality=Row vector (2-D)
      settings: AttributesFormatString=%<OutputDimensionality>
  V1 : Constant  Value=V1  VectorParams1D=off
      settings: AttributesFormatString=%<Value>\n%<VectorParams1D>
  V2 : Constant  Value=V2  VectorParams1D=off  OutDataTypeStr=single
      settings: AttributesFormatString=%<Value>\n%<VectorParams1D>
  Vector Concatenate : Concatenate  NumInputs=3  Mode=Multidimensional array
      settings: AttributesFormatString=%<Mode>
  onetofour : Selector  IndexOptions=Index vector (dialog)  Indices=[1:nRed+3]  OutputSizes=1
  onetothree : Selector  IndexOptions=Index vector (dialog)  Indices=[1:nRed+2]  OutputSizes=1
  sixtonine : Selector  IndexOptions=Index vector (dialog)  Indices=[nRed+5:nRed+8]  OutputSizes=1
  ten : Selector  IndexOptions=Index vector (dialog)  Indices=[nRed+9]  OutputSizes=1
  twelve : Selector  IndexOptions=Index vector (dialog)  Indices=[nRed+11]  OutputSizes=1
  boutput : Outport  OutDataTypeStr=single
  wires:
  Vector Concatenate/1 -> Gain7/1
  ten/1 -> Add/1
  sixtonine/1 -> MathFunction/1
  onetothree/1 -> MathFunction1/1
  Product3/1 -> Add/2
  Product4/1 -> Add1/2
  uinput/1 -> Reshape_input/1
  onetofour/1 -> MathFunction2/1
  Add1/1 -> Vector Concatenate/3
  Add/1 -> Vector Concatenate/2
  twelve/1 -> Add1/1
  V1/1 -> Product3/1
  V2/1 -> Product4/1
  Gain7/1 -> boutput/1
  Reshape_input/1 -> twelve/1, onetofour/1, ten/1, onetothree/1, sixtonine/1
  MathFunction/1 -> Vector Concatenate/1
  MathFunction1/1 -> Product3/2
  MathFunction2/1 -> Product4/2

== system KD_cl_harness_cl_ouports_added/ctrl_rb_explicit_20140220_v6_simp/HQPKWIK_V6/x0_calculation ==
  uinput : Inport
  " 1" : Selector  IndexOptions=Index vector (dialog)  Indices=[1:nRed+2]  OutputSizes=1
  Gain : Gain  Gain=2
  Gain1 : Gain  Gain=-1
  Math Function2 : Math  Operator=transpose  SaturateOnIntegerOverflow=on
  Product1 : Product  Multiplication=Matrix(*)  RndMeth=Zero
  Product6 : Product  Multiplication=Matrix(*)  RndMeth=Zero
  Q_inv : Constant  Value=Q_inv  VectorParams1D=off  OutDataTypeStr=single
      settings: AttributesFormatString=%<Value>\n%<VectorParams1D>
  Reshape_input : Reshape  OutputDimensionality=Row vector (2-D)
      settings: AttributesFormatString=%<OutputDimensionality>
  f_mat : Constant  Value=f_mat  VectorParams1D=off  OutDataTypeStr=single
      settings: AttributesFormatString=%<Value>\n%<VectorParams1D>
  xout : Outport
  c : Outport  Port=2
  wires:
  uinput/1 -> Reshape_input/1
  Gain/1 -> " 1"/1
  " 1"/1 -> Product6/1
  f_mat/1 -> Product6/2
  Q_inv/1 -> Gain1/1
  Product1/1 -> xout/1
  Product6/1 -> Math Function2/1
  Gain1/1 -> Product1/1
  Math Function2/1 -> c/1, Product1/2
  Reshape_input/1 -> Gain/1

== system KD_cl_harness_cl_ouports_added/ctrl_rb_explicit_20140220_v6_simp/calc_y_constraints/If_Action_Subsystem ==
  In1 : Inport
  In2 : Inport  Port=2
  Action Port : ActionPort  ActionType=then
  Sum6 : Sum  Inputs=|++
  Out1 : Outport  InitialOutput=250
  wires:
  Sum6/1 -> Out1/1
  In1/1 -> Sum6/1
  In2/1 -> Sum6/2

== system KD_cl_harness_cl_ouports_added/ctrl_rb_explicit_20140220_v6_simp/egr_est/custom_filter ==
  Input : Inport
  Data Store Read1 : DataStoreRead  DataStoreName=man_tuneFiltalpha
  Data Store Read8 : DataStoreRead  DataStoreName=man_tuneFiltalpha
  Delay1 : Delay  DelayLength=1  InitialCondition=0
  Product1 : Product  Inputs=**  RndMeth=Zero
  Product2 : Product  Inputs=**  RndMeth=Zero
  Saturation1 : Saturate  UpperLimit=1  LowerLimit=0
      settings: AttributesFormatString=%<LowerLimit>\n%<UpperLimit>
  Saturation4 : Saturate  UpperLimit=1  LowerLimit=0
      settings: AttributesFormatString=%<LowerLimit>\n%<UpperLimit>
  Sum1 : Sum  Inputs=+-|
  Sum11 : Sum  Inputs=++|
  man_tuneFiltalpha : Gain
  man_tuneFiltalpha1 : Gain
  zero1 : Constant  OutDataTypeStr=single  SampleTime=sample_time
      settings: AttributesFormatString=%<Value>\n%<SampleTime>
  Output : Outport  OutDataTypeStr=single
  sat_out-25 : Outport  Port=2
  sat_out-26 : Outport  Port=3
  wires:
  Input/1 -> Product1/2
  Delay1/1 -> Product2/1
  Data Store Read8/1 -> man_tuneFiltalpha1/1
  Product2/1 -> Sum11/1
  Sum1/1 -> Product1/1
  Data Store Read1/1 -> man_tuneFiltalpha/1
  Saturation4/1 -> Sum1/2
  Saturation1/1 -> Product2/2
  Product1/1 -> Sum11/2
  zero1/1 -> Sum1/1
  Sum11/1 -> Output/1, Delay1/1
  man_tuneFiltalpha/1 -> Saturation4/1, sat_out-26/1
  man_tuneFiltalpha1/1 -> Saturation1/1, sat_out-25/1

== system KD_cl_harness_cl_ouports_added/ctrl_rb_explicit_20140220_v6_simp/egr_est/interp ==
  valve : Inport
  MAF : Inport  Port=2
  Wcyl : Inport  Port=3
  Product : Product  RndMeth=Zero
  Product1 : Product  RndMeth=Zero
  Sum : Sum  Inputs=-+|
  Sum1 : Sum  Inputs=++|
  interp : Lookup  InputValues=[0 15]  Table=[0 1]  LookUpMeth=Interpolation-Use End Values
      settings: AttributesFormatString=%<LookUpMeth>\n%<InputValues>
  one : Constant  OutDataTypeStr=single  SampleTime=sample_time
      settings: AttributesFormatString=%<Value>\n%<SampleTime>
  Wcylhat : Outport
  wires:
  valve/1 -> interp/1
  Wcyl/1 -> Product/1
  interp/1 -> Product/2, Sum/1
  one/1 -> Sum/2
  Sum/1 -> Product1/1
  MAF/1 -> Product1/2
  Product1/1 -> Sum1/2
  Product/1 -> Sum1/1
  Sum1/1 -> Wcylhat/1

== system KD_cl_harness_cl_ouports_added/ctrl_rb_explicit_20140220_v6_simp/input_processing/pex_filter ==
  pexh_ecu : Inport
  Gain1 : Gain  Gain=sysll.c  Multiplication=Matrix(K*u) (u vector)  OutDataTypeStr=single
      settings: AttributesFormatString=%<Multiplication>
  Gain2 : Gain  Gain=sysll.a  Multiplication=Matrix(K*u) (u vector)  OutDataTypeStr=single
      settings: AttributesFormatString=%<Multiplication>
  Gain3 : Gain  Gain=sysll.b  Multiplication=Matrix(K*u) (u vector)  OutDataTypeStr=single
      settings: AttributesFormatString=%<Multiplication>
  Sum : Sum  Inputs=++|
  Unit Delay5 : UnitDelay  InitialCondition=[0;0]  SampleTime=-1
      settings: AttributesFormatString=%<X0>
  pex_filt : Outport  OutDataTypeStr=single
  wires:
  Gain1/1 -> pex_filt/1
  Gain3/1 -> Sum/1
  pexh_ecu/1 -> Gain3/1
  Unit Delay5/1 -> Gain2/1
  Sum/1 -> Gain1/1, Unit Delay5/1
  Gain2/1 -> Sum/2

== system KD_cl_harness_cl_ouports_added/ctrl_rb_explicit_20140220_v6_simp/ntremap/custom_filter ==
  Input : Inport
  Delay1 : Delay  DelayLength=1  InitialCondition=0
      settings: AttributesFormatString=%<vinit>
  Product1 : Product  Inputs=**  RndMeth=Zero
  Product2 : Product  Inputs=**  RndMeth=Zero
  Saturation1 : Saturate  UpperLimit=1  LowerLimit=0
      settings: AttributesFormatString=%<LowerLimit>\n%<UpperLimit>
  Saturation4 : Saturate  UpperLimit=1  LowerLimit=0
      settings: AttributesFormatString=%<LowerLimit>\n%<UpperLimit>
  Sum1 : Sum  Inputs=+-|
  Sum11 : Sum  Inputs=++|
  filt : Constant  Value=c_filt  OutDataTypeStr=single  SampleTime=sample_time
      settings: AttributesFormatString=%<Value>\n%<SampleTime>
  filt1 : Constant  Value=c_filt  OutDataTypeStr=single  SampleTime=sample_time
      settings: AttributesFormatString=%<Value>\n%<SampleTime>
  one : Constant  OutDataTypeStr=single  SampleTime=sample_time
      settings: AttributesFormatString=%<Value>\n%<SampleTime>
  Output : Outport  OutDataTypeStr=single
  sat_out-27 : Outport  Port=2
  sat_out-28 : Outport  Port=3
  wires:
  Input/1 -> Product1/2
  Delay1/1 -> Product2/1
  filt/1 -> Saturation1/1, sat_out-27/1
  Product2/1 -> Sum11/1
  Sum1/1 -> Product1/1
  filt1/1 -> Saturation4/1, sat_out-28/1
  Saturation4/1 -> Sum1/2
  Saturation1/1 -> Product2/2
  Product1/1 -> Sum11/2
  one/1 -> Sum1/1
  Sum11/1 -> Output/1, Delay1/1

== system KD_cl_harness_cl_ouports_added/ctrl_rb_explicit_20140220_v6_simp/ntremap/remap_wt_to_map ==
  In1 : Inport
  In2 : Inport  Port=2
  In3 : Inport  Port=3
  In4 : Inport  Port=4
  In5 : Inport  Port=5
  In6 : Inport  Port=6
  In7 : Inport  Port=7
  Divide1 : Product  Inputs=/*
  LookupTable_2D1 : Lookup2D  RowIndex=c_vwcompdes  ColumnIndex=c_vpout  Table=c_compmap
      settings: AttributesFormatString=%<RowIndex>\n%<ColumnIndex>\n%<Table>
  Saturation2 : Saturate  UpperLimit=50  LowerLimit=8
      settings: AttributesFormatString=%<LowerLimit>\n%<UpperLimit>
  Saturation3 : Saturate  UpperLimit=300  LowerLimit=100
      settings: AttributesFormatString=%<LowerLimit>\n%<UpperLimit>
  Sum1 : Sum  Inputs=++|  OutDataTypeStr=single
  Sum3 : Sum  Inputs=-+|
  ThrottleModel1 : Subsystem
  Unit Delay : UnitDelay  InitialCondition=7  SampleTime=-1
      settings: AttributesFormatString=%<X0>
  Unit Delay1 : UnitDelay  InitialCondition=7  SampleTime=-1
      settings: AttributesFormatString=%<X0>
  While Iterator : WhileIterator  MaxIters=30
  conversion to radpers2 : Gain  Gain=c_rpmtoradpers
  conversion to radpers3 : Gain  Gain=single(1/1000)
  pincomp1 : Constant  Value=c_pincomp  OutDataTypeStr=single  SampleTime=-1
      settings: AttributesFormatString=%<Value>\n%<SampleTime>
  pincomp2 : Constant  OutDataTypeStr=single  SampleTime=-1
      settings: AttributesFormatString=%<Value>\n%<SampleTime>
  scaling1 : Gain  Gain=1000
  pinv : Outport
  wtinv : Outport  Port=2
  sat_out-29 : Outport  Port=3
  sat_out-30 : Outport  Port=4
  sat_out-45 : Outport  Port=5
  sat_out-46 : Outport  Port=6
  sat_out-58 : Outport  Port=7
  sat_out-59 : Outport  Port=8
  sat_out-60 : Outport  Port=9
  sat_out-61 : Outport  Port=10
  sat_out-62 : Outport  Port=11
  sat_out-63 : Outport  Port=12
  sat_out-64 : Outport  Port=13
  sat_out-65 : Outport  Port=14
  out-17 : Outport  Port=15
  out-28 : Outport  Port=16
  wires:
  Saturation3/1 -> Unit Delay1/1
  Saturation2/1 -> Unit Delay/1
  In7/1 -> While Iterator/2
  pincomp2/1 -> While Iterator/1
  Sum1/1 -> Saturation3/1, pinv/1, scaling1/1, sat_out-30/1
  Unit Delay1/1 -> Sum1/1
  Sum3/1 -> Sum1/2
  Unit Delay/1 -> Sum3/1
  In4/1 -> Sum3/2
  conversion to radpers3/1 -> wtinv/1, Saturation2/1, sat_out-29/1
  In6/1 -> ThrottleModel1/5(wegrthr)
  In5/1 -> ThrottleModel1/4(Tamb_K)
  In3/1 -> LookupTable_2D1/1
  In2/1 -> ThrottleModel1/2(Ne_rpm)
  In1/1 -> ThrottleModel1/1(TA_deg)
  conversion to radpers2/1 -> conversion to radpers3/1
  scaling1/1 -> ThrottleModel1/3(Pim_Pa)
  ThrottleModel1/1(p_pre_throttle) -> Divide1/2
  LookupTable_2D1/1 -> conversion to radpers2/1
  pincomp1/1 -> Divide1/1
  Divide1/1 -> LookupTable_2D1/2
  ThrottleModel1/2(sat_out-45) -> sat_out-45/1
  ThrottleModel1/3(sat_out-46) -> sat_out-46/1
  ThrottleModel1/4(sat_out-58) -> sat_out-58/1
  ThrottleModel1/5(sat_out-59) -> sat_out-59/1
  ThrottleModel1/6(sat_out-60) -> sat_out-60/1
  ThrottleModel1/7(sat_out-61) -> sat_out-61/1
  ThrottleModel1/8(sat_out-62) -> sat_out-62/1
  ThrottleModel1/9(sat_out-63) -> sat_out-63/1
  ThrottleModel1/10(sat_out-64) -> sat_out-64/1
  ThrottleModel1/11(sat_out-65) -> sat_out-65/1
  ThrottleModel1/12(out-17) -> out-17/1
  ThrottleModel1/13(out-28) -> out-28/1

== system KD_cl_harness_cl_ouports_added/ctrl_rb_explicit_20140220_v6_simp/pex_estimator/WhileIteratorSubsystem ==
  valvez : Inport
  Ne_rpm : Inport  Port=2
  map : Inport  Port=3
  wger : Inport  Port=4
  tico : Inport  Port=5
  pex_filt : Inport  Port=6
  While : Inport  Port=7
  pexz : Inport  Port=8
  Constant10 : Constant  Value=SVR_EGR_exhat.Beta
  Constant11 : Constant  Value=SVR_EGR_exhat.SV2
  Constant12 : Constant  Value=SVR_EGR_exhat.SV1
  Constant13 : Constant  Value=const_exhat.k
  Constant14 : Constant  Value=SVR_EGR_exhat.arg
  Constant7 : Constant  Value=const_exhat.Pcab
  Constant8 : Constant  Value=const_exhat.Tcab
  Gain10 : Gain  Gain=c_p01
      settings: AttributesFormatString=%<Gain>
  Gain11 : Gain  Gain=c_4400inv
      settings: AttributesFormatString=%<Gain>
  Mux14 : Mux  Inputs=2
  Saturation4 : Saturate  UpperLimit=c_inf  LowerLimit=c_80
      settings: AttributesFormatString=%<LowerLimit>\n%<UpperLimit>
  Saturation_Dynamic2 : simulink/Discontinuities/Saturation Dynamic  OutMin=[]  OutMax=[]  OutDataTypeStr=Inherit: Same as second input  OutDataType=fixdt(1, 16)  OutScaling=2^-10  DoSatur=off
  Sum14 : Sum  Inputs=++|
  While_Ioop : WhileIterator
  newton : Subsystem
  pexmax1 : Constant  Value=1000  OutDataTypeStr=single  SampleTime=-1
      settings: AttributesFormatString=%<Value>\n%<SampleTime>
  unity2 : Constant  OutDataTypeStr=single  SampleTime=-1
      settings: AttributesFormatString=%<Value>\n%<SampleTime>
  y_cons4 : Constant  OutDataTypeStr=boolean  SampleTime=-1
      settings: AttributesFormatString=%<Value>\n%<SampleTime>
  pex : Outport
  dwdp : Outport  Port=2
  pex_limited : Outport  Port=3
  sat_out-31 : Outport  Port=4
  sat_out-32 : Outport  Port=5
  sat_out-33 : Outport  Port=6
  sat_out-34 : Outport  Port=7
  sat_out-35 : Outport  Port=8
  sat_out-36 : Outport  Port=9
  sat_out-47 : Outport  Port=10
  sat_out-48 : Outport  Port=11
  sat_out-49 : Outport  Port=12
  sat_out-50 : Outport  Port=13
  sat_out-51 : Outport  Port=14
  sat_out-52 : Outport  Port=15
  sat_out-53 : Outport  Port=16
  sat_out-54 : Outport  Port=17
  sat_out-55 : Outport  Port=18
  sat_out-56 : Outport  Port=19
  sat_out-57 : Outport  Port=20
  wires:
  y_cons4/1 -> While_Ioop/1
  Constant14/1 -> newton/5(arg)
  Constant12/1 -> newton/3(SV1)
  Constant10/1 -> newton/2(Beta)
  Gain11/1 -> Mux14/2
  Gain10/1 -> Mux14/1
  Mux14/1 -> newton/1(u)
  Constant7/1 -> newton/9(pcab)
  Constant8/1 -> newton/10(tcab)
  Constant13/1 -> newton/12(k)
  newton/1(pexkp1) -> pex/1, Saturation_Dynamic2/2
  Saturation_Dynamic2/1 -> pex_limited/1
  unity2/1 -> Sum14/1
  Sum14/1 -> Saturation_Dynamic2/3
  pexmax1/1 -> Saturation_Dynamic2/1
  Constant11/1 -> newton/4(SV2)
  Saturation4/1 -> Sum14/2
  valvez/1 -> Gain10/1
  Ne_rpm/1 -> Gain11/1
  map/1 -> newton/7(pin), Saturation4/1, sat_out-31/1
  wger/1 -> newton/8(wegrmeas)
  newton/2(dwdp) -> dwdp/1
  tico/1 -> newton/11(tex)
  pex_filt/1 -> newton/13(pex_ecu)
  While/1 -> While_Ioop/2
  pexz/1 -> newton/6(pex)
  newton/3(sat_out-32) -> sat_out-32/1
  newton/4(sat_out-33) -> sat_out-33/1
  newton/5(sat_out-34) -> sat_out-34/1
  newton/6(sat_out-35) -> sat_out-35/1
  newton/7(sat_out-36) -> sat_out-36/1
  newton/8(sat_out-47) -> sat_out-47/1
  newton/9(sat_out-48) -> sat_out-48/1
  newton/10(sat_out-49) -> sat_out-49/1
  newton/11(sat_out-50) -> sat_out-50/1
  newton/12(sat_out-51) -> sat_out-51/1
  newton/13(sat_out-52) -> sat_out-52/1
  newton/14(sat_out-53) -> sat_out-53/1
  newton/15(sat_out-54) -> sat_out-54/1
  newton/16(sat_out-55) -> sat_out-55/1
  newton/17(sat_out-56) -> sat_out-56/1
  newton/18(sat_out-57) -> sat_out-57/1
